simulink model "render_puma_560"  (Simulink 10.2)
settings: Solver=VariableStepAuto  StartTime=0.0  StopTime=0.1  RelTol=1e-3
undefined symbols (not defined in the file): q
libraries: vrlib x1
settings Model: Creator=jasper  LastModifiedBy=jasper
settings DataIOCC: SaveFormat=Dataset  SignalLoggingSaveFormat=Dataset  ReturnWorkspaceOutputs=on
settings OptimizationCC: LifeSpan=auto
settings DebuggingCC: UnderspecifiedInitializationDetection=Simplified  MergeDetectMultiDrivingBlocksExec=error  FcnCallInpInsideContextMsg=error  SFUnexpectedBacktrackingDiag=error  SFNoUnconditionalDefaultTransitionDiag=error  SFExecutionAtInitializationDiag=warning  ArithmeticOperatorsInVariantConditions=error
settings HardwareCC: ProdBitPerPointer=64  ProdBitPerSizeT=64  ProdBitPerPtrDiffT=64  ProdLargestAtomicFloat=Float  ProdIntDivRoundTo=Zero  ProdEndianess=LittleEndian  ProdWordSize=64  ProdHWDeviceType=Intel->x86-64 (Windows64)
settings ModelReferenceCC: PropagateSignalLabelsOutOfModel=on
settings SFSimCC: SimUseLocalCustomCode=on  CustomCodeUndefinedFunction=FilterOut
settings RTWCC: RTWUseLocalCustomCode=on
settings CodeAppCC: StateflowObjectComments=off
settings GRTTargetCC: TargetLangStandard=C99 (ISO)  CombineOutputUpdateFcns=on  GRTInterface=off
settings ConfigComp: CovMetricSettings=dwe  CovSaveCumulativeToWorkspaceVar=off  CovSaveSingleToWorkspaceVar=off  CovExternalEMLEnable=on

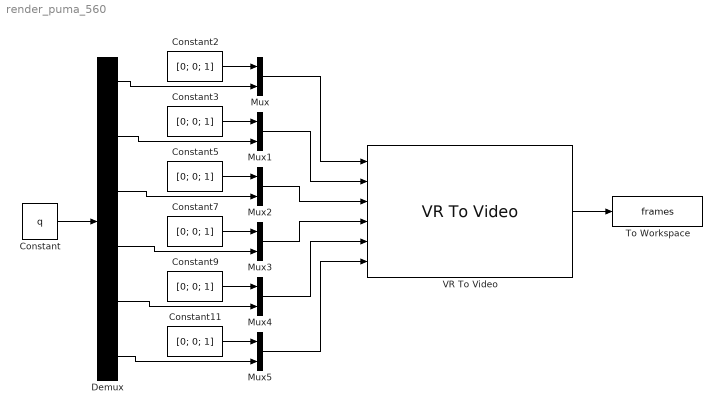
== system render_puma_560 ==
  Constant : Constant  Value=q
  Constant{2..3,5,7,9,11} (6 alike) : Constant  Value=[0; 0; 1]
  Demux : Demux  Outputs=6
  Mux{,1..5} (6 alike) : Mux  Inputs=2
  To Workspace : ToWorkspace  VariableName=frames  SaveFormat=Timeseries  SampleTime=-1
  VR To Video : vrlib/VR To Video  InstantiateOnLoad=on  SampleTime=0.1  ViewEnable=on  RemoteChange=off  RemoteView=off  FieldsWritten=l1_REVOLUTE.rotation.4.1.1.double#l2_REVOLUTE.rotation.4.1.1.double#l3_REVOLUTE.rotation.4.1.1.double#l4_REVOLUTE.rotation.4.1.1.double#l5_REVOLUTE.rotation.4.1.1.double#l6_REVOLUTE.rotation.4.1.1.double  WorldFileName=puma_560_dh.x3d  AutoView=off  VideoDimensions=[2160 3840]  AllowVariableSize=off
      settings: SourceProductBaseCode=SL
  wires:
  Constant2/1 -> Mux/1
  Constant3/1 -> Mux1/1
  Constant5/1 -> Mux2/1
  Constant7/1 -> Mux3/1
  Constant9/1 -> Mux4/1
  Constant11/1 -> Mux5/1
  Mux/1 -> VR To Video/1
  Mux1/1 -> VR To Video/2
  Mux2/1 -> VR To Video/3
  Mux5/1 -> VR To Video/6
  Mux4/1 -> VR To Video/5
  Mux3/1 -> VR To Video/4
  Demux/1 -> Mux/2
  Demux/2 -> Mux1/2
  Demux/3 -> Mux2/2
  Demux/4 -> Mux3/2
  Demux/5 -> Mux4/2
  Demux/6 -> Mux5/2
  Constant/1 -> Demux/1
  VR To Video/1 -> To Workspace/1
